simulink model "sistema_fisico"  (R2019a)
settings: Solver=VariableStepAuto  StartTime=0.0  StopTime=10.0  RelTol=1e-3
undefined symbols (not defined in the file or in its folder): b_eqh, ih, J_eqh, Rd
settings Model: Creator=Facundo  LastModifiedBy=Facundo

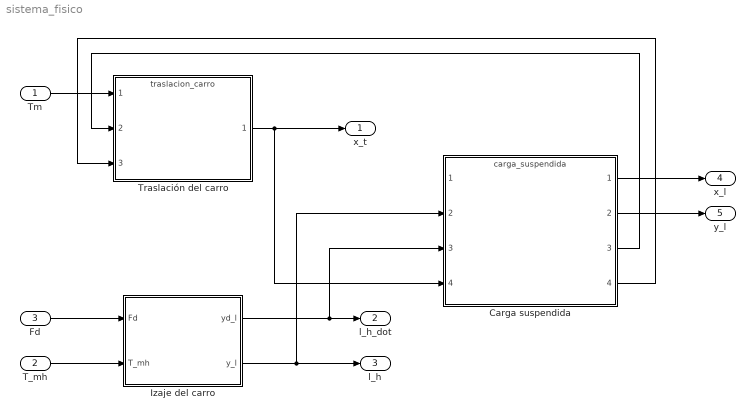
== system sistema_fisico ==
  Tm : Inport
  T_mh : Inport  Port=2
  Fd : Inport  Port=3
  Carga suspendida : ModelReference  ModelNameDialog=carga_suspendida.slx  SimulationMode=Normal  ModelReferenceVersion=1.8
  Izaje del carro : Subsystem
  Traslación del carro : ModelReference  ModelNameDialog=traslacion_carro  SimulationMode=Normal  ModelReferenceVersion=1.7
  x_t : Outport
  l_h_dot : Outport  Port=2
  l_h : Outport  Port=3
  x_l : Outport  Port=4
  y_l : Outport  Port=5
  wires:
  Traslación del carro/1 -> Carga suspendida/4, x_t/1
  Tm/1 -> Traslación del carro/1
  Fd/1 -> Izaje del carro/1(Fd)
  T_mh/1 -> Izaje del carro/2(T_mh)
  Izaje del carro/1(yd_l) -> Carga suspendida/3, l_h_dot/1
  Izaje del carro/2(y_l) -> Carga suspendida/2, l_h/1
  Carga suspendida/1 -> x_l/1
  Carga suspendida/2 -> y_l/1
  Carga suspendida/3 -> Traslación del carro/2
  Carga suspendida/4 -> Traslación del carro/3

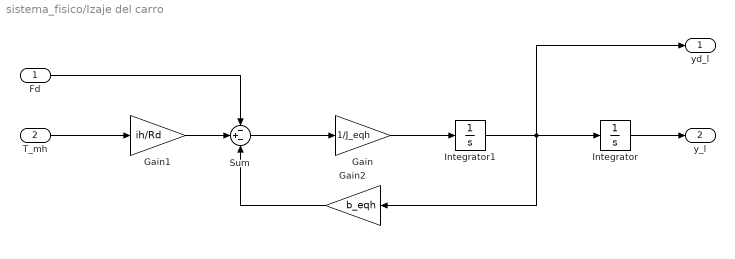
== system sistema_fisico/Izaje del carro ==
  Fd : Inport
  T_mh : Inport  Port=2
  Gain : Gain  Gain=1/J_eqh
  Gain1 : Gain  Gain=ih/Rd
  Gain2 : Gain  Gain=b_eqh
  Integrator : Integrator
  Integrator1 : Integrator
  Sum : Sum  Inputs=-+-
  yd_l : Outport
  y_l : Outport  Port=2
  wires:
  Gain/1 -> Integrator1/1
  Integrator1/1 -> yd_l/1, Gain2/1, Integrator/1
  Gain2/1 -> Sum/3
  Sum/1 -> Gain/1
  Gain1/1 -> Sum/2
  Integrator/1 -> y_l/1
  Fd/1 -> Sum/1
  T_mh/1 -> Gain1/1
